simulink model "MOSSE_HDL_HIL_final"  (Simulink 8.1)
settings: Solver=FixedStepDiscrete  SolverMode=SingleTasking  StartTime=0.0  StopTime=20*30*640*360  RelTol=1e-3
InitFcn:
  | %% DSPBuilder Start
  | alt_dspbuilder_update_model(bdroot)
  | %% DSPBuilder End
  | K_shift = 4
  | 
  | ksize = 5
  | load('Gauss_coeff.mat')
  | tic
StopFcn:
  | % r = rcount.Data(:,:);
  | % w = wcount.Data(:,:);
  | % d = dout.Data(:,:);
  | % ir = read.Data(:,:);
  | % iw = write.Data(:,:);
  | % z = double([ir iw d r w]');
  | %logic_analyzer
  | toc
undefined symbols (not defined in the file or in its folder): gray, psr, source_1, source_2, State_Machine, State_Transition_Table1
libraries: allblocks_alteradspbuilder2 x75, hdldemolib x2, dspsigattribs x2, dspmtrx3 x2, visionsinks x1, visiontextngfix x1, dspvision x1
(part 1 of 2)
settings Model: FPTRunName=FPA_Reference  Creator=minimal  LastModifiedBy=minimal
settings DataIOCC: SignalLoggingSaveFormat=Dataset
settings OptimizationCC: ExpressionDepthLimit=128
settings DebuggingCC: FcnCallInpInsideContextMsg=EnableAllAsError
settings HardwareCC: ProdHWDeviceType=ASIC/FPGA->ASIC/FPGA  TargetIntDivRoundTo=Zero  TargetEndianess=LittleEndian  TargetHWDeviceType=MATLAB Host  ProdEqTarget=off
settings GRTTargetCC: CombineOutputUpdateFcns=on  GRTInterface=off

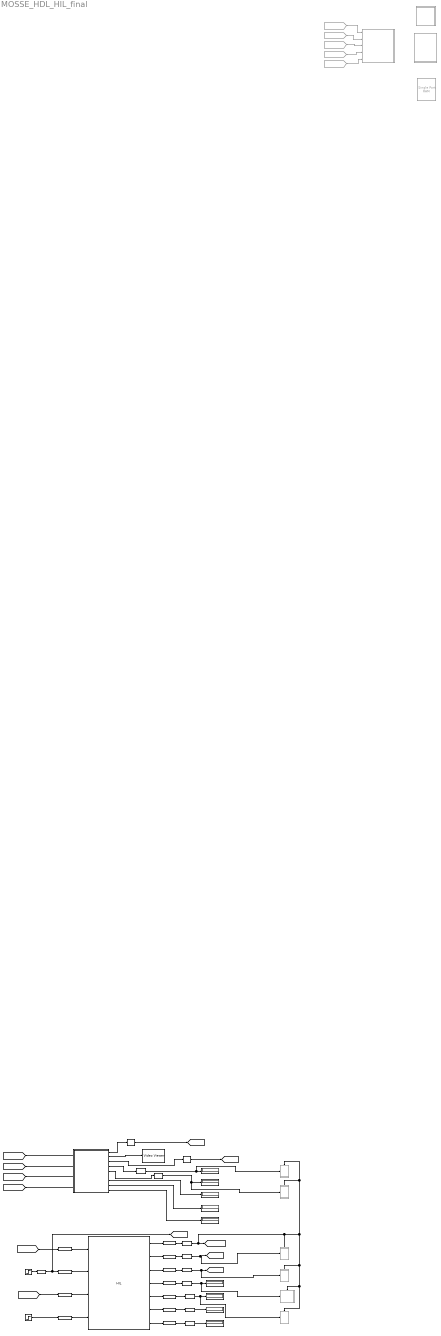
== system MOSSE_HDL_HIL_final ==
  Comp_Shift_Finish : allblocks_alteradspbuilder2/Output  iofile=d:\Project\AutoTracking\model\MOSSE_work\MOSSE_model\test\tb_MOSSE_HDL_HIL_final\MOSSE%5FHDL%5FHIL%5Ffinal_Comp%5FShift%5FFinish.capture  BusType=Single Bit  bwl=8  bwr=0  externalType=Simulink Fixed Point Type  PORTTYPE=Output  allowFloatingPointOverride=on  logOutputs=off
  DSP_Builder_Compute_PSR : Subsystem  Commented=on
  DSP_Builder_Compute_Shift : Subsystem  Commented=on
  Data Type Conversion{4,6..7,10} (4 alike) : DataTypeConversion  OutDataTypeStr=boolean
  Data Type Conversion11 : DataTypeConversion  OutDataTypeStr=int8
  Data Type Conversion12 : DataTypeConversion  OutDataTypeStr=int8
  Data Type Conversion13 : DataTypeConversion  OutDataTypeStr=uint16
  Data Type Conversion5 : DataTypeConversion  OutDataTypeStr=int16
  Data Type Conversion8 : DataTypeConversion  OutDataTypeStr=uint16
  Data Type Conversion9 : DataTypeConversion  OutDataTypeStr=uint16
  Delay2 : Delay  DelayLength=1  InitialCondition=0  SampleTime=1
  Delay3 : Delay  DelayLength=1  InitialCondition=0  SampleTime=1
  Display{,1..2,6} (4 alike) : Display
  Dx : allblocks_alteradspbuilder2/Output  iofile=d:\Project\AutoTracking\model\MOSSE_work\MOSSE_model\test\tb_MOSSE_HDL_HIL_final\MOSSE%5FHDL%5FHIL%5Ffinal_Dx.capture  BusType=Signed Integer  bwl=8  bwr=0  externalType=Simulink Fixed Point Type  PORTTYPE=Output  allowFloatingPointOverride=on  logOutputs=off
  Dy : allblocks_alteradspbuilder2/Output  iofile=d:\Project\AutoTracking\model\MOSSE_work\MOSSE_model\test\tb_MOSSE_HDL_HIL_final\MOSSE%5FHDL%5FHIL%5Ffinal_Dy.capture  BusType=Signed Integer  bwl=8  bwr=0  externalType=Simulink Fixed Point Type  PORTTYPE=Output  allowFloatingPointOverride=on  logOutputs=off
  Enable_Tracking : allblocks_alteradspbuilder2/Input  iofile=d:\Project\AutoTracking\model\MOSSE_work\MOSSE_model\test\tb_MOSSE_HDL_HIL_final\MOSSE%5FHDL%5FHIL%5Ffinal_Enable%5FTracking.salt  BusType=Single Bit  bwl=8  bwr=0  SpecifyClock=off  PORTTYPE=Input  externalType=Inferred  allowFloatingPointOverride=on  logOutputs=off
  Enable_Write : allblocks_alteradspbuilder2/Input  iofile=d:\Project\AutoTracking\model\MOSSE_work\MOSSE_model\test\tb_MOSSE_HDL_HIL_final\MOSSE%5FHDL%5FHIL%5Ffinal_Enable%5FWrite.salt  BusType=Single Bit  bwl=8  bwr=0  SpecifyClock=off  PORTTYPE=Input  externalType=Inferred  allowFloatingPointOverride=on  logOutputs=off
  From38 : From  Commented=on  GotoTag=source_enb
  From39 : From  Commented=on  GotoTag=source1_enb
  From40 : From  Commented=on  GotoTag=source_control
  From41 : From  Commented=on  GotoTag=source_count_enb
  From42 : From  Commented=on  GotoTag=source_count_rst
  HIL : allblocks_alteradspbuilder2/HIL  entityName=MOSSE_HDL_code_gen_final  inNames=Input_image enable_tracking enable_write reset  inBwls="8  1  1  1  1  1"  inBwrs="0  0  0  0  0  0"  inTypes=u b b b  inDelayed="0  0  0  0"  outNames=comp_shift_finish dx dy max_index psr psr_check psr_finish  outBwls="1   8   8  13  16   1   1"  outBwrs="0  0  0  0  0  0  0"  outTypes=b s s u s b b  resetNames=aclr  InputCount=6  InputNames=Clock Input_image aclr enable_tracking enable_write reset  InputWidth="1  8  1  1  1  1"  InputRepresentation="0  0  0  0  0  0"  InputExport="2  0  3  0  0  0"  InputFPP="0  0  0  0  0  0"  OutputCount=7  OutputNames=comp_shift_finish dx dy max_index psr psr_check psr_finish  OutputWidth="1   8   8  13  16   1   1"  OutputRepresentation="0  1  1  0  1  0  0"  OutputExport="0  0  0  0  0  0  0"  OutputFPP="0  0  0  0  0  0  0"  JtagCable=1  JtagDevice=1  BurstMode=on  BurstLength=512  FrameMode=off  SOP=0  OutValid=0  QuartusProject=D:\Project\AutoTracking\model\MOSSE_work\MOSSE_model\test\MOSSE_HDL_code_gen_final_dspbuilder\MOSSE_HDL_code_gen_final.qpf  HilNewConfig=off  ClockPinLocation=K17  ClockPinSource=0  HilDeviceOnBoard=EP4CE115F29C7  DR_length=56  dspbuilder_reset=on  SLD_NODE_INFO=5167554  AssertSclrBeforeSimulation=1  SampleTime=0  dspb_ver=0  ResetLevel=0  JtagCableName=USB-Blaster [USB-0]  JtagDeviceName=@1: EP3C120/EP4CE115 (0x020F70DD)  ClockNames=Clock
  IFFT_res : hdldemolib/Single Port RAM  Commented=on  ram_size=12  dout_type=New data
  Input_image : allblocks_alteradspbuilder2/Input  iofile=d:\Project\AutoTracking\model\MOSSE_work\MOSSE_model\test\tb_MOSSE_HDL_HIL_final\MOSSE%5FHDL%5FHIL%5Ffinal_Input%5Fimage.salt  BusType=Unsigned Integer  bwl=8  bwr=0  SpecifyClock=off  PORTTYPE=Input  externalType=Inferred  allowFloatingPointOverride=on  logOutputs=off
  Reset : allblocks_alteradspbuilder2/Input  iofile=d:\Project\AutoTracking\model\MOSSE_work\MOSSE_model\test\tb_MOSSE_HDL_HIL_final\MOSSE%5FHDL%5FHIL%5Ffinal_Reset.salt  BusType=Single Bit  bwl=8  bwr=0  SpecifyClock=off  PORTTYPE=Input  externalType=Inferred  allowFloatingPointOverride=on  logOutputs=off
  Source : Subsystem  Commented=on
  Step : Step  Before=1  After=0  SampleTime=0
  Step1 : Step  SampleTime=0
  Subsystem : Subsystem  Commented=on
  Subsystem1 : Subsystem  Commented=on
  Subsystem2 : Subsystem  Commented=on
  Subsystem3 : Subsystem  Commented=on
  Subsystem4 : Subsystem  Commented=on
  Subsystem5 : Subsystem  Commented=on
  Video Viewer2 : visionsinks/Video Viewer  inputType=Obsolete7b  imagePorts=One multidimensional signal  useColorMap=off  colormapValue=gray(256)  specRange=off  minInputVal=0  maxInputVal=255  FigPos=[321 948 1218 708]  AxisZoom=on  trueSizedOnce=off  OpenAtMdlStart=on  DefaultConfigurationName=vipscopes.VideoViewerScopeCfg
  Video_TestBench1 : Subsystem
  addr_x : Display
  addr_y : Display
  frame_num : Display
  max_index : allblocks_alteradspbuilder2/Output  iofile=d:\Project\AutoTracking\model\MOSSE_work\MOSSE_model\test\tb_MOSSE_HDL_HIL_final\MOSSE%5FHDL%5FHIL%5Ffinal_max%5Findex.capture  BusType=Unsigned Integer  bwl=13  bwr=0  externalType=Simulink Fixed Point Type  PORTTYPE=Output  allowFloatingPointOverride=on  logOutputs=off
  "psr " : allblocks_alteradspbuilder2/Output  iofile=d:\Project\AutoTracking\model\MOSSE_work\MOSSE_model\test\tb_MOSSE_HDL_HIL_final\MOSSE%5FHDL%5FHIL%5Ffinal_psr%0A.capture  BusType=Signed Integer  bwl=16  bwr=0  externalType=Simulink Fixed Point Type  PORTTYPE=Output  allowFloatingPointOverride=on  logOutputs=off
  psr_check : allblocks_alteradspbuilder2/Output  iofile=d:\Project\AutoTracking\model\MOSSE_work\MOSSE_model\test\tb_MOSSE_HDL_HIL_final\MOSSE%5FHDL%5FHIL%5Ffinal_psr%5Fcheck.capture  BusType=Single Bit  bwl=8  bwr=0  externalType=Simulink Fixed Point Type  PORTTYPE=Output  allowFloatingPointOverride=on  logOutputs=off
  psr_finish : allblocks_alteradspbuilder2/Output  iofile=d:\Project\AutoTracking\model\MOSSE_work\MOSSE_model\test\tb_MOSSE_HDL_HIL_final\MOSSE%5FHDL%5FHIL%5Ffinal_psr%5Ffinish.capture  BusType=Single Bit  bwl=8  bwr=0  externalType=Simulink Fixed Point Type  PORTTYPE=Output  allowFloatingPointOverride=on  logOutputs=off
  x : Display
  y : Display
  wires:
  From40/1 -> Source/1(source_control)
  From38/1 -> Source/2(source_enb)
  From42/1 -> Source/3(source_count_rst)
  From41/1 -> Source/4(source_count_enb)
  From39/1 -> Source/5(source1_enb)
  Data Type Conversion10/1 -> Subsystem/Enable, Subsystem2/Enable, Subsystem3/Enable, Subsystem1/Enable, Subsystem5/Enable, Subsystem4/Enable, [comp_shift_finish]
  Step/1 -> Reset/1
  Input_image/1 -> HIL/1
  Reset/1 -> HIL/4
  HIL/1 -> Comp_Shift_Finish/1
  HIL/2 -> Dx/1
  HIL/3 -> Dy/1
  [input_image] -> Input_image/1
  HIL/4 -> max_index/1
  HIL/6 -> psr_check/1
  Video_TestBench1/2(video_viewer) -> Video Viewer2/1
  Video_TestBench1/1(enable_write) -> Delay2/1
  Video_TestBench1/3(serialized_data) -> Delay3/1
  Delay3/1 -> [input_image]
  Delay2/1 -> [enable_write]
  [enable_tracking] -> Video_TestBench1/1(en)
  [comp_shift_finish] -> Video_TestBench1/4(comp_shift_finish)
  [dx] -> Video_TestBench1/2(dx)
  [dy] -> Video_TestBench1/3(dy)
  "psr "/1 -> Data Type Conversion5/1
  Data Type Conversion5/1 -> Subsystem2/1(psr), Display1/1
  psr_check/1 -> Data Type Conversion4/1
  Data Type Conversion4/1 -> Display/1
  psr_finish/1 -> Data Type Conversion6/1
  Data Type Conversion6/1 -> Display2/1
  HIL/7 -> psr_finish/1
  HIL/5 -> "psr "/1
  Video_TestBench1/7(frame_num) -> frame_num/1
  Data Type Conversion8/1 -> Subsystem4/1(addr_x), x/1
  Data Type Conversion9/1 -> Subsystem5/1(addr_y), y/1
  Video_TestBench1/8(addr_x) -> addr_x/1
  Video_TestBench1/9(addr_y) -> addr_y/1
  Enable_Tracking/1 -> HIL/2
  Data Type Conversion7/1 -> [enable_tracking], Enable_Tracking/1
  Step1/1 -> Data Type Conversion7/1
  [enable_write] -> Enable_Write/1
  Enable_Write/1 -> HIL/3
  Video_TestBench1/4(x) -> Data Type Conversion8/1
  Video_TestBench1/5(y) -> Data Type Conversion9/1
  Comp_Shift_Finish/1 -> Data Type Conversion10/1
  Data Type Conversion11/1 -> [dx], Subsystem/1(dx)
  Dx/1 -> Data Type Conversion11/1
  Dy/1 -> Data Type Conversion12/1
  Data Type Conversion12/1 -> [dy], Subsystem1/1(dy)
  max_index/1 -> Data Type Conversion13/1
  Data Type Conversion13/1 -> Display6/1, Subsystem3/1(max_index)

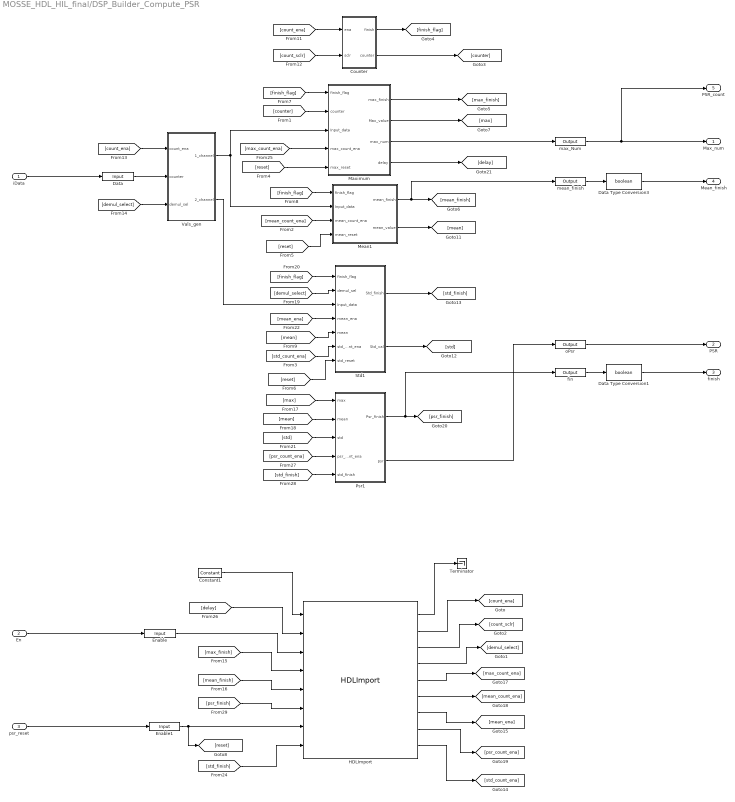
== system MOSSE_HDL_HIL_final/DSP_Builder_Compute_PSR ==
  iData : Inport
  En : Inport  Port=2
  psr_reset : Inport  Port=3
  Constant1 : allblocks_alteradspbuilder2/Constant  mask_cst=1  BusType=Single Bit  bwl=8  bwr=0  roundMode=Truncate  satMode=Wrap  SpecifyClock=off  allowFloatingPointOverride=on  logOutputs=off  logFile=d:\Project\AutoTracking\model\MOSSE_work\MOSSE_model\MOSSE_Final_models\tb_MOSSE_HDL_final\MOSSE%5FHDL%5Ffinal_DSP%5FBuilder%5FCompute%5FPSR_Constant1.fixedpointlog
  Counter : Subsystem
  Data : allblocks_alteradspbuilder2/Input  iofile=d:\Project\AutoTracking\model\MOSSE_work\MOSSE_model\MOSSE_Final_models\tb_MOSSE_HDL_final\MOSSE%5FHDL%5Ffinal_DSP%5FBuilder%5FCompute%5FPSR_Data.salt  BusType=Signed Integer  bwl=16  bwr=0  SpecifyClock=off  PORTTYPE=Input  externalType=Inferred  allowFloatingPointOverride=on  logOutputs=off
  Data Type Conversion1 : DataTypeConversion  OutDataTypeStr=boolean
  Data Type Conversion3 : DataTypeConversion  OutDataTypeStr=boolean
  Enable : allblocks_alteradspbuilder2/Input  iofile=d:\Project\AutoTracking\model\MOSSE_work\MOSSE_model\MOSSE_Final_models\tb_MOSSE_HDL_final\MOSSE%5FHDL%5Ffinal_DSP%5FBuilder%5FCompute%5FPSR_Enable.salt  BusType=Single Bit  bwl=16  bwr=0  SpecifyClock=off  PORTTYPE=Input  externalType=Inferred  allowFloatingPointOverride=on  logOutputs=off
  Enable1 : allblocks_alteradspbuilder2/Input  iofile=d:\Project\AutoTracking\model\MOSSE_work\MOSSE_model\MOSSE_Final_models\tb_MOSSE_HDL_final\MOSSE%5FHDL%5Ffinal_DSP%5FBuilder%5FCompute%5FPSR_Enable1.salt  BusType=Single Bit  bwl=16  bwr=0  SpecifyClock=off  PORTTYPE=Input  externalType=Inferred  allowFloatingPointOverride=on  logOutputs=off
  HDLImport : allblocks_alteradspbuilder2/HDLImport  entityName=State_Machine_import  inNames=clk_enable delay enable_in max_finish mean_finish psr_finish reset std_finish  inBwls=1 1 1 1 1 1 1 1  inBwrs="0  0  0  0  0  0  0  0"  inTypes=b b b b b b b b  inDelayed="0  0  0  0  0  0  0  0"  outNames=ce_out count_ena count_sclr demul_select max_count_ena mean_count_ena mean_ena psr_count_ena std_count_ena  outBwls=1 1 1 1 1 1 1 1 1  outBwrs="0  0  0  0  0  0  0  0  0"  outTypes=b b b b b b b b b  xmlmapfile=C:\altera\13.0\quartus\dsp_builder\lib\SimgenCMap.xml  vofile=DSPBuilder_MOSSE_HDL_final_import\State_Machine.vo  src_file=psr\State_Machine.v;psr\State_Transition_Table1.v;  TopLevelName=State_Machine  UseQPF=0  n_input_port=8  n_output_port=9  array_clocks=clk  use_systemC_model=off  is_megacore=off  use_dynamic_feedthrough_data=off  use_alphabetical_port_ordering=on  allowFloatingPointOverride=off
  Maximum : Subsystem
  Mean1 : Subsystem
  Psr1 : Subsystem
  Std1 : Subsystem
  Terminator : Terminator
  Vals_gen : Subsystem
  fin : allblocks_alteradspbuilder2/Output  iofile=d:\Project\AutoTracking\model\MOSSE_work\MOSSE_model\MOSSE_Final_models\tb_MOSSE_HDL_final\MOSSE%5FHDL%5Ffinal_DSP%5FBuilder%5FCompute%5FPSR_fin.capture  BusType=Single Bit  bwl=32  bwr=0  externalType=Simulink Fixed Point Type  PORTTYPE=Output  allowFloatingPointOverride=on  logOutputs=off
  max_Num : allblocks_alteradspbuilder2/Output  iofile=d:\Project\AutoTracking\model\MOSSE_work\MOSSE_model\MOSSE_Final_models\tb_MOSSE_HDL_final\MOSSE%5FHDL%5Ffinal_DSP%5FBuilder%5FCompute%5FPSR_max%5FNum.capture  BusType=Signed Integer  bwl=16  bwr=0  externalType=Simulink Fixed Point Type  PORTTYPE=Output  allowFloatingPointOverride=on  logOutputs=off
  mean_finish : allblocks_alteradspbuilder2/Output  iofile=d:\Project\AutoTracking\model\MOSSE_work\MOSSE_model\MOSSE_Final_models\tb_MOSSE_HDL_final\MOSSE%5FHDL%5Ffinal_DSP%5FBuilder%5FCompute%5FPSR_mean%5Ffinish.capture  BusType=Single Bit  bwl=16  bwr=0  externalType=Simulink Fixed Point Type  PORTTYPE=Output  allowFloatingPointOverride=on  logOutputs=off
  oPsr : allblocks_alteradspbuilder2/Output  iofile=d:\Project\AutoTracking\model\MOSSE_work\MOSSE_model\MOSSE_Final_models\tb_MOSSE_HDL_final\MOSSE%5FHDL%5Ffinal_DSP%5FBuilder%5FCompute%5FPSR_oPsr.capture  BusType=Signed Integer  bwl=32  bwr=0  externalType=Simulink Fixed Point Type  PORTTYPE=Output  allowFloatingPointOverride=on  logOutputs=off
  Max_num : Outport
  PSR : Outport  Port=2
  finish : Outport  Port=3
  Mean_finish : Outport  Port=4
  PSR_count : Outport  Port=5
  wires:
  [demul_select] -> Std1/2(demul_sel)
  Data/1 -> Vals_gen/2(counter)
  [demul_select] -> Vals_gen/3(demul_sel)
  Vals_gen/2(2_channel) -> Std1/3(Input_data)
  [finish_flag] -> Std1/1(finish_flag)
  Std1/1(Std_finish) -> [std_finish]
  Mean1/2(mean_value) -> [mean]
  max_Num/1 -> PSR_count/1, Max_num/1
  Maximum/2(Max_value) -> [max]
  [mean] -> Std1/5(mean)
  [mean_ena] -> Std1/4(mean_ena)
  [max] -> Psr1/1(max)
  Maximum/4(delay) -> [delay]
  HDLImport/1 -> Terminator/1
  Constant1/1 -> HDLImport/1
  [psr_finish] -> HDLImport/6
  [std_finish] -> HDLImport/8
  [mean_finish] -> HDLImport/5
  [max_finish] -> HDLImport/4
  [delay] -> HDLImport/2
  Mean1/1(mean_finish) -> mean_finish/1, [mean_finish]
  oPsr/1 -> PSR/1
  [count_ena] -> Vals_gen/1(count_ena)
  Psr1/1(Psr_finish) -> fin/1, [psr_finish]
  Vals_gen/1(1_channel) -> Maximum/3(Input_data), Mean1/2(Input_data)
  [mean_count_ena] -> Mean1/3(mean_count_ena)
  Counter/1(finish) -> [finish_flag]
  Maximum/1(max_finish) -> [max_finish]
  [counter] -> Maximum/2(counter)
  [finish_flag] -> Maximum/1(finish_flag)
  [finish_flag] -> Mean1/1(finish_flag)
  [count_ena] -> Counter/1(ena)
  [count_sclr] -> Counter/2(sclr)
  [std_finish] -> Psr1/5(std_finish)
  Psr1/2(psr) -> oPsr/1
  [mean] -> Psr1/2(mean)
  [std] -> Psr1/3(std)
  Std1/2(Std_val) -> [std]
  [std_count_ena] -> Std1/6(std_count_ena)
  [psr_count_ena] -> Psr1/4(psr_count_ena)
  [max_count_ena] -> Maximum/4(max_count_ena)
  HDLImport/3 -> [count_sclr]
  HDLImport/2 -> [count_ena]
  HDLImport/6 -> [mean_count_ena]
  Enable/1 -> HDLImport/3
  HDLImport/4 -> [demul_select]
  HDLImport/5 -> [max_count_ena]
  HDLImport/7 -> [mean_ena]
  HDLImport/8 -> [psr_count_ena]
  HDLImport/9 -> [std_count_ena]
  Counter/2(counter) -> [counter]
  En/1 -> Enable/1
  iData/1 -> Data/1
  psr_reset/1 -> Enable1/1
  Enable1/1 -> [reset], HDLImport/7
  mean_finish/1 -> Data Type Conversion3/1
  fin/1 -> Data Type Conversion1/1
  Data Type Conversion1/1 -> finish/1
  Data Type Conversion3/1 -> Mean_finish/1
  [reset] -> Maximum/5(max_reset)
  [reset] -> Mean1/4(mean_reset)
  [reset] -> Std1/7(std_reset)
  Maximum/3(max_num) -> max_Num/1

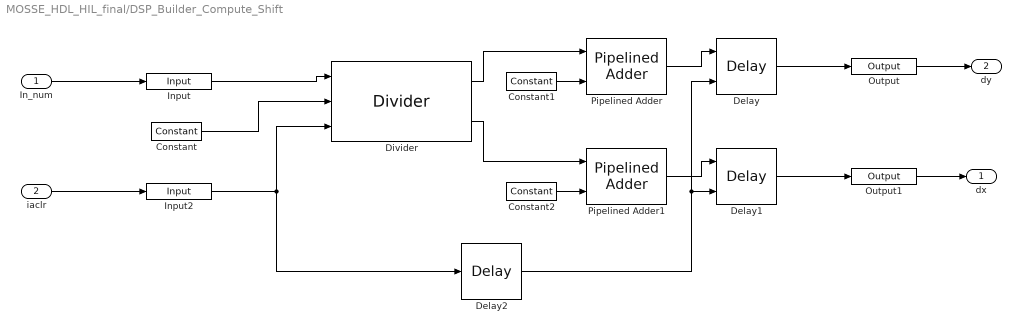
== system MOSSE_HDL_HIL_final/DSP_Builder_Compute_Shift ==
  In_num : Inport
  iaclr : Inport  Port=2
  Constant : allblocks_alteradspbuilder2/Constant  mask_cst=64  BusType=Unsigned Integer  bwl=8  bwr=0  roundMode=Truncate  satMode=Wrap  SpecifyClock=off  allowFloatingPointOverride=on  logOutputs=off  logFile=C:\Workspace\Autotracking\MOSSE_model\tb_MOSSE_HDL_final\MOSSE%5FHDL%5Ffinal_DSP%5FBuilder%5FCompute%5FShift_Constant.fixedpointlog
  Constant1 : allblocks_alteradspbuilder2/Constant  mask_cst=31  BusType=Signed Integer  bwl=8  bwr=0  roundMode=Truncate  satMode=Wrap  SpecifyClock=off  allowFloatingPointOverride=on  logOutputs=off  logFile=C:\Workspace\Autotracking\MOSSE_model\tb_MOSSE_HDL_final\MOSSE%5FHDL%5Ffinal_DSP%5FBuilder%5FCompute%5FShift_Constant1.fixedpointlog
  Constant2 : allblocks_alteradspbuilder2/Constant  mask_cst=32  BusType=Signed Integer  bwl=8  bwr=0  roundMode=Truncate  satMode=Wrap  SpecifyClock=off  allowFloatingPointOverride=on  logOutputs=off  logFile=C:\Workspace\Autotracking\MOSSE_model\tb_MOSSE_HDL_final\MOSSE%5FHDL%5Ffinal_DSP%5FBuilder%5FCompute%5FShift_Constant2.fixedpointlog
  Delay : allblocks_alteradspbuilder2/Delay  pipeline=1  pipeline_display=1  ClockPhase=1  use_ena=off  use_sclr=on  allowFloatingPointOverride=on  logOutputs=off  logFile=C:\Workspace\Autotracking\MOSSE_model\tb_MOSSE_HDL_final\MOSSE%5FHDL%5Ffinal_DSP%5FBuilder%5FCompute%5FShift_Delay.fixedpointlog  use_init=off  reset_value=1
  Delay1 : allblocks_alteradspbuilder2/Delay  pipeline=1  pipeline_display=1  ClockPhase=1  use_ena=off  use_sclr=on  allowFloatingPointOverride=on  logOutputs=off  logFile=C:\Workspace\Autotracking\MOSSE_model\tb_MOSSE_HDL_final\MOSSE%5FHDL%5Ffinal_DSP%5FBuilder%5FCompute%5FShift_Delay1.fixedpointlog  use_init=off  reset_value=1
  Delay2 : allblocks_alteradspbuilder2/Delay  pipeline=1  pipeline_display=1  ClockPhase=1  use_ena=off  use_sclr=off  allowFloatingPointOverride=on  logOutputs=off  logFile=C:\Workspace\Autotracking\MOSSE_model\tb_MOSSE_HDL_final\MOSSE%5FHDL%5Ffinal_DSP%5FBuilder%5FCompute%5FShift_Delay2.fixedpointlog  use_init=off  reset_value=1
  Divider : allblocks_alteradspbuilder2/Divider  BusType=Unsigned Integer  bwl=12  bwr=0  pipeline=1  pipeline_display=1  use_ena=off  use_aclr=on
  Input : allblocks_alteradspbuilder2/Input  iofile=C:\Workspace\Autotracking\MOSSE_model\tb_MOSSE_HDL_final\MOSSE%5FHDL%5Ffinal_DSP%5FBuilder%5FCompute%5FShift_Input.salt  BusType=Unsigned Integer  bwl=12  bwr=0  SpecifyClock=off  PORTTYPE=Input  externalType=Inferred  allowFloatingPointOverride=on  logOutputs=off
  Input2 : allblocks_alteradspbuilder2/Input  iofile=C:\Workspace\Autotracking\MOSSE_model\tb_MOSSE_HDL_final\MOSSE%5FHDL%5Ffinal_DSP%5FBuilder%5FCompute%5FShift_Input2.salt  BusType=Single Bit  bwl=12  bwr=0  SpecifyClock=off  PORTTYPE=Input  externalType=Inferred  allowFloatingPointOverride=on  logOutputs=off
  Output : allblocks_alteradspbuilder2/Output  iofile=C:\Workspace\Autotracking\MOSSE_model\tb_MOSSE_HDL_final\MOSSE%5FHDL%5Ffinal_DSP%5FBuilder%5FCompute%5FShift_Output.capture  BusType=Signed Integer  bwl=8  bwr=0  externalType=Simulink Fixed Point Type  PORTTYPE=Output  allowFloatingPointOverride=on  logOutputs=off
  Output1 : allblocks_alteradspbuilder2/Output  iofile=C:\Workspace\Autotracking\MOSSE_model\tb_MOSSE_HDL_final\MOSSE%5FHDL%5Ffinal_DSP%5FBuilder%5FCompute%5FShift_Output1.capture  BusType=Signed Integer  bwl=8  bwr=0  externalType=Simulink Fixed Point Type  PORTTYPE=Output  allowFloatingPointOverride=on  logOutputs=off
  Pipelined Adder : allblocks_alteradspbuilder2/Pipelined Adder  BusType=Signed Integer  bwl=12  bwr=0  pipeline=0  pipeline_display=0  AddSubDirection=SUB  use_cin=off  use_ovl=off  use_addsub=off  use_ena=off  use_aclr=off  or_aclr_inputs=on
  Pipelined Adder1 : allblocks_alteradspbuilder2/Pipelined Adder  BusType=Signed Integer  bwl=12  bwr=0  pipeline=0  pipeline_display=0  AddSubDirection=SUB  use_cin=off  use_ovl=off  use_addsub=off  use_ena=off  use_aclr=off  or_aclr_inputs=on
  dx : Outport
  dy : Outport  Port=2
  wires:
  Input/1 -> Divider/1
  Constant/1 -> Divider/2
  In_num/1 -> Input/1
  Output1/1 -> dx/1
  Output/1 -> dy/1
  Divider/1 -> Pipelined Adder/1
  Constant2/1 -> Pipelined Adder1/2
  Pipelined Adder/1 -> Delay/1
  Delay/1 -> Output/1
  Pipelined Adder1/1 -> Delay1/1
  Delay1/1 -> Output1/1
  Divider/2 -> Pipelined Adder1/1
  iaclr/1 -> Input2/1
  Input2/1 -> Delay2/1, Divider/3
  Constant1/1 -> Pipelined Adder/2
  Delay2/1 -> Delay/2, Delay1/2

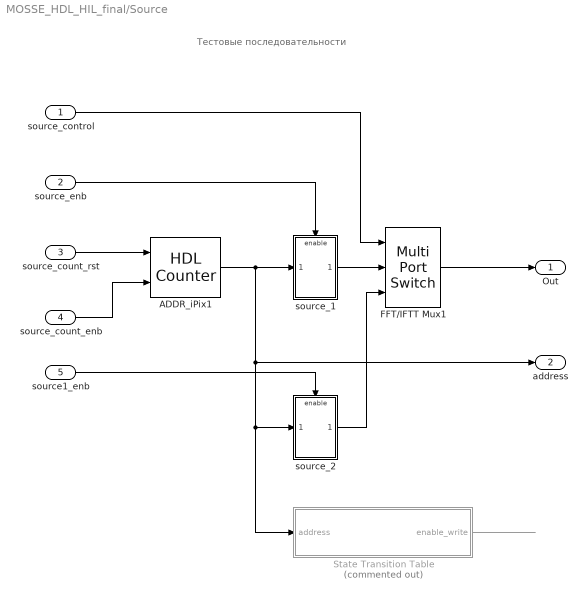
== system MOSSE_HDL_HIL_final/Source ==
  note: Тестовые последовательности
  source_control : Inport
  source_enb : Inport  Port=2
  source_count_rst : Inport  Port=3
  source_count_enb : Inport  Port=4
  source1_enb : Inport  Port=5
  ADDR_iPix1 : hdldemolib/HDL Counter  CountType=Free running  CountInit=0  CountStep=1  CountMax=100  CountFromType=Initial value  CountFrom=0  CountResetPort=on  CountLoadPort=off  CountEnbPort=on  CountDirPort=off  CountDataType=Unsigned  CountWordLen=32  CountFracLen=0  CountSampTime=1
  FFT/IFTT Mux1 : MultiPortSwitch  DataPortOrder=Zero-based contiguous  Inputs=2  zeroidx=on  OutDataTypeStr=fixdt(1,24,0)  SampleTime=1
  State Transition Table : State Transition Table  Commented=on  TreatAsAtomicUnit=on
  source_1 : Subsystem
  source_2 : Subsystem
  Out : Outport
  address : Outport  Port=2
  wires:
  ADDR_iPix1/1 -> address/1, State Transition Table/1(address), source_2/1(In1), source_1/1(In1)
  source_enb/1 -> source_1/Enable
  source1_enb/1 -> source_2/Enable
  source_count_enb/1 -> ADDR_iPix1/2
  FFT/IFTT Mux1/1 -> Out/1
  source_count_rst/1 -> ADDR_iPix1/1
  source_1/1(Out1) -> FFT/IFTT Mux1/2
  source_control/1 -> FFT/IFTT Mux1/1
  source_2/1(Out1) -> FFT/IFTT Mux1/3
  State Transition Table/1(enable_write) -> ?

== system MOSSE_HDL_HIL_final/Subsystem ==
  dx : Inport
  Enable : EnablePort
  To Workspace : ToWorkspace  VariableName=dx  SampleTime=-1
  wires:
  dx/1 -> To Workspace/1

== system MOSSE_HDL_HIL_final/Subsystem1 ==
  dy : Inport
  Enable : EnablePort
  To Workspace : ToWorkspace  VariableName=dy  SampleTime=-1
  wires:
  dy/1 -> To Workspace/1

== system MOSSE_HDL_HIL_final/Subsystem2 ==
  psr : Inport
  Enable : EnablePort
  To Workspace : ToWorkspace  VariableName=psr  SampleTime=-1
  wires:
  psr/1 -> To Workspace/1

== system MOSSE_HDL_HIL_final/Subsystem3 ==
  max_index : Inport
  Enable : EnablePort
  To Workspace : ToWorkspace  VariableName=max_index  SampleTime=-1
  wires:
  max_index/1 -> To Workspace/1

== system MOSSE_HDL_HIL_final/Subsystem4 ==
  addr_x : Inport
  Enable : EnablePort
  To Workspace : ToWorkspace  VariableName=addr_x  SampleTime=-1
  wires:
  addr_x/1 -> To Workspace/1

== system MOSSE_HDL_HIL_final/Subsystem5 ==
  addr_y : Inport
  Enable : EnablePort
  To Workspace : ToWorkspace  VariableName=addr_y  SampleTime=-1
  wires:
  addr_y/1 -> To Workspace/1

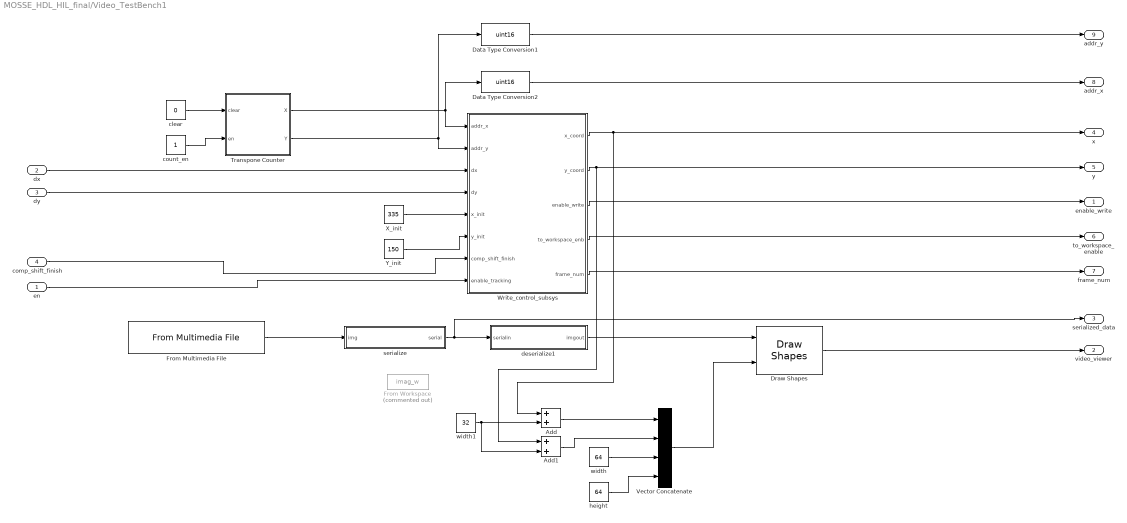
== system MOSSE_HDL_HIL_final/Video_TestBench1 ==
  en : Inport
  dx : Inport  Port=2
  dy : Inport  Port=3
  comp_shift_finish : Inport  Port=4
  Add : Sum  AccumDataTypeStr=uint16
  Add1 : Sum  AccumDataTypeStr=uint16
  Data Type Conversion1 : DataTypeConversion  OutDataTypeStr=uint16
  Data Type Conversion2 : DataTypeConversion  OutDataTypeStr=uint16
  Draw Shapes : visiontextngfix/Draw Shapes  shape=Rectangles  fill=off  fillClrSource=Specify via dialog  display=User-specified value  intensity=200  color=[255]  opacity=0.6  viewport=Entire image  antialiasing=off  inType=Obsolete  imagePorts=One multidimensional signal  prodOutputMode=Binary point scaling  prodOutputWordLength=32  prodOutputFracLength=14  memoryMode=Specify word length  memoryWordLength=16  memoryFracLength=15  roundingMode=Floor  overflowMode=off
  From Workspace : FromWorkspace  Commented=on  VariableName=imag_w  SampleTime=1
  From Multimedia File : dspvision/From Multimedia File  inputFilename=D:\Project\AutoTracking\model\MOSSE_work\MOSSE_model\test\test_video_2.avi  loop=on  numPlays=inf  outputStreams=Video only  videoDataType=uint8  audioDataType=int16  inheritSampleTime=off  userDefinedSampleTime=640*360  noAudioOutput=off  isIntensityVideo=off  fourcc=Intensity  colorVideoFormat=One multidimensional signal  outputEOF=off  dataOrg=Column-major  audioFrameSize=1024  computeAudioFrameSize=off  outSamplingMode=Sample based
  Transpone Counter : MATLAB Function
  Vector Concatenate : Concatenate  NumInputs=4
  Write_control_subsys : Subsystem
  X_init : Constant  Value=335  OutDataTypeStr=uint16
  Y_init : Constant  Value=150  OutDataTypeStr=uint16
  clear : Constant  Value=0  OutDataTypeStr=boolean
  count_en : Constant  OutDataTypeStr=boolean
  deserialize1 : Subsystem
  height : Constant  Value=64  OutDataTypeStr=uint16
  serialize : Subsystem
  width : Constant  Value=64  OutDataTypeStr=uint16
  width1 : Constant  Value=32  OutDataTypeStr=uint16
  enable_write : Outport
  video_viewer : Outport  Port=2
  serialized_data : Outport  Port=3
  x : Outport  Port=4
  y : Outport  Port=5
  to_workspace_enable : Outport  Port=6
  frame_num : Outport  Port=7
  addr_x : Outport  Port=8
  addr_y : Outport  Port=9
  wires:
  From Multimedia File/1 -> serialize/1(img)
  deserialize1/1(imgout) -> Draw Shapes/1
  serialize/1(serial) -> deserialize1/1(serialin), serialized_data/1
  Transpone Counter/2(Y) -> Write_control_subsys/2(addr_y), Data Type Conversion1/1
  Transpone Counter/1(X) -> Write_control_subsys/1(addr_x), Data Type Conversion2/1
  count_en/1 -> Transpone Counter/2(en)
  clear/1 -> Transpone Counter/1(clear)
  en/1 -> Write_control_subsys/8(enable_tracking)
  Draw Shapes/1 -> video_viewer/1
  width/1 -> Vector Concatenate/3
  height/1 -> Vector Concatenate/4
  Vector Concatenate/1 -> Draw Shapes/2
  Add1/1 -> Vector Concatenate/2
  Add/1 -> Vector Concatenate/1
  Data Type Conversion1/1 -> addr_y/1
  Data Type Conversion2/1 -> addr_x/1
  width1/1 -> Add/2, Add1/2
  Write_control_subsys/1(x_coord) -> x/1, Add/1
  Write_control_subsys/2(y_coord) -> y/1, Add1/1
  dx/1 -> Write_control_subsys/3(dx)
  X_init/1 -> Write_control_subsys/5(x_init)
  dy/1 -> Write_control_subsys/4(dy)
  comp_shift_finish/1 -> Write_control_subsys/7(comp_shift_finish)
  Write_control_subsys/3(enable_write) -> enable_write/1
  Write_control_subsys/4(to_workspace_enb) -> to_workspace_enable/1
  Write_control_subsys/5(frame_num) -> frame_num/1
  Y_init/1 -> Write_control_subsys/6(y_init)

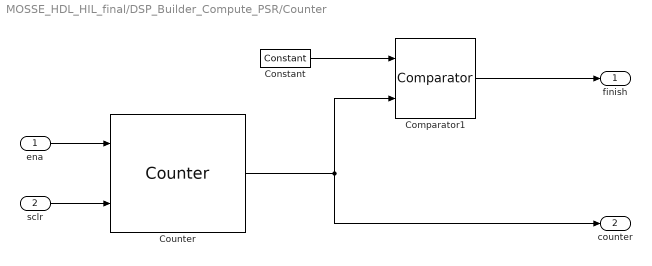
== system MOSSE_HDL_HIL_final/DSP_Builder_Compute_PSR/Counter ==
  ena : Inport
  sclr : Inport  Port=2
  Comparator1 : allblocks_alteradspbuilder2/Comparator  direction=a == b  pipeline_display=0  allowFloatingPointOverride=on  logOutputs=off  logFile=d:\Project\AutoTracking\model\MOSSE_work\MOSSE_model\MOSSE_Final_models\tb_MOSSE_HDL_final\MOSSE%5FHDL%5Ffinal_DSP%5FBuilder%5FCompute%5FPSR_Counter_Comparator1.fixedpointlog
  Constant : allblocks_alteradspbuilder2/Constant  mask_cst=4095  BusType=Unsigned Integer  bwl=16  bwr=0  roundMode=Truncate  satMode=Wrap  SpecifyClock=off  allowFloatingPointOverride=on  logOutputs=off  logFile=d:\Project\AutoTracking\model\MOSSE_work\MOSSE_model\MOSSE_Final_models\tb_MOSSE_HDL_final\MOSSE%5FHDL%5Ffinal_DSP%5FBuilder%5FCompute%5FPSR_Counter_Constant.fixedpointlog
  Counter : allblocks_alteradspbuilder2/Counter  BusType=Unsigned Integer  bwl=16  bwr=0  use_modulo=on  modulo=4100  SpecifyClock=off  direction=Increment  use_sload=off  use_sset=off  svalue=1  use_clk_ena=off  use_ena=on  use_sclr=on  pipeline_display=1
  finish : Outport
  counter : Outport  Port=2
  wires:
  Constant/1 -> Comparator1/1
  Counter/1 -> counter/1, Comparator1/2
  Comparator1/1 -> finish/1
  sclr/1 -> Counter/2
  ena/1 -> Counter/1

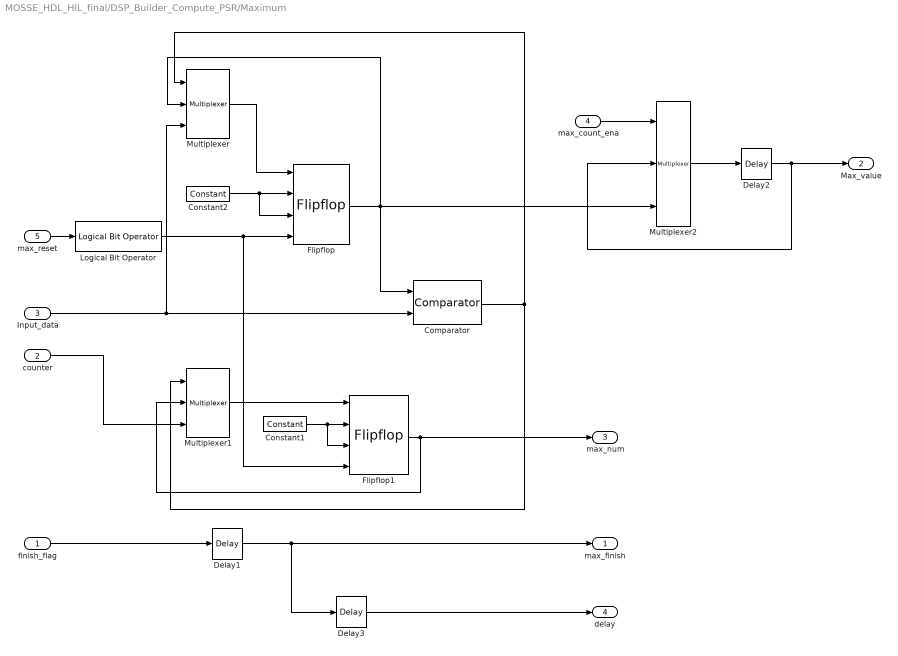
== system MOSSE_HDL_HIL_final/DSP_Builder_Compute_PSR/Maximum ==
  finish_flag : Inport
  counter : Inport  Port=2
  Input_data : Inport  Port=3
  max_count_ena : Inport  Port=4
  max_reset : Inport  Port=5
  Comparator : allblocks_alteradspbuilder2/Comparator  direction=a < b  pipeline_display=0  allowFloatingPointOverride=on  logOutputs=off  logFile=d:\Project\AutoTracking\model\MOSSE_work\MOSSE_model\MOSSE_Final_models\tb_MOSSE_HDL_final\MOSSE%5FHDL%5Ffinal_DSP%5FBuilder%5FCompute%5FPSR_Maximum_Comparator.fixedpointlog
  Constant1 : allblocks_alteradspbuilder2/Constant  mask_cst=1  BusType=Single Bit  bwl=24  bwr=0  roundMode=Truncate  satMode=Wrap  SpecifyClock=off  allowFloatingPointOverride=on  logOutputs=off  logFile=d:\Project\AutoTracking\model\MOSSE_work\MOSSE_model\MOSSE_Final_models\tb_MOSSE_HDL_final\MOSSE%5FHDL%5Ffinal_DSP%5FBuilder%5FCompute%5FPSR_Maximum_Constant1.fixedpointlog
  Constant2 : allblocks_alteradspbuilder2/Constant  mask_cst=1  BusType=Single Bit  bwl=24  bwr=0  roundMode=Truncate  satMode=Wrap  SpecifyClock=off  allowFloatingPointOverride=on  logOutputs=off  logFile=d:\Project\AutoTracking\model\MOSSE_work\MOSSE_model\MOSSE_Final_models\tb_MOSSE_HDL_final\MOSSE%5FHDL%5Ffinal_DSP%5FBuilder%5FCompute%5FPSR_Maximum_Constant2.fixedpointlog
  Delay1 : allblocks_alteradspbuilder2/Delay  pipeline=2  pipeline_display=2  ClockPhase=1  use_ena=off  use_sclr=off  allowFloatingPointOverride=on  logOutputs=off  logFile=d:\Project\AutoTracking\model\MOSSE_work\MOSSE_model\MOSSE_Final_models\tb_MOSSE_HDL_final\MOSSE%5FHDL%5Ffinal_DSP%5FBuilder%5FCompute%5FPSR_Maximum_Delay1.fixedpointlog  use_init=off  reset_value=1
  Delay2 : allblocks_alteradspbuilder2/Delay  pipeline=1  pipeline_display=1  ClockPhase=1  use_ena=off  use_sclr=off  allowFloatingPointOverride=on  logOutputs=off  logFile=d:\Project\AutoTracking\model\MOSSE_work\MOSSE_model\MOSSE_Final_models\tb_MOSSE_HDL_final\MOSSE%5FHDL%5Ffinal_DSP%5FBuilder%5FCompute%5FPSR_Maximum_Delay2.fixedpointlog  use_init=off  reset_value=1
  Delay3 : allblocks_alteradspbuilder2/Delay  pipeline=1  pipeline_display=1  ClockPhase=1  use_ena=off  use_sclr=off  allowFloatingPointOverride=on  logOutputs=off  logFile=d:\Project\AutoTracking\model\MOSSE_work\MOSSE_model\MOSSE_Final_models\tb_MOSSE_HDL_final\MOSSE%5FHDL%5Ffinal_DSP%5FBuilder%5FCompute%5FPSR_Maximum_Delay3.fixedpointlog  use_init=off  reset_value=1
  Flipflop : allblocks_alteradspbuilder2/Flipflop  mode=DFFE  BusType=Signed Integer  bwl=16  bwr=2  pipeline_display=1
  Flipflop1 : allblocks_alteradspbuilder2/Flipflop  mode=DFFE  BusType=Signed Integer  bwl=16  bwr=2  pipeline_display=1
  Logical Bit Operator : allblocks_alteradspbuilder2/Logical Bit Operator  LogicalOperator=NOT  user_inputs=2  pipeline_display=0
  Multiplexer : allblocks_alteradspbuilder2/Multiplexer  numInputs=2  pipeline=0  oneHot=off  pipeline_display=0  use_ena=off  use_aclr=off  allowFloatingPointOverride=on  logOutputs=off  logFile=d:\Project\AutoTracking\model\MOSSE_work\MOSSE_model\MOSSE_Final_models\tb_MOSSE_HDL_final\MOSSE%5FHDL%5Ffinal_DSP%5FBuilder%5FCompute%5FPSR_Maximum_Multiplexer.fixedpointlog
  Multiplexer1 : allblocks_alteradspbuilder2/Multiplexer  numInputs=2  pipeline=0  oneHot=off  pipeline_display=0  use_ena=off  use_aclr=off  allowFloatingPointOverride=on  logOutputs=off  logFile=d:\Project\AutoTracking\model\MOSSE_work\MOSSE_model\MOSSE_Final_models\tb_MOSSE_HDL_final\MOSSE%5FHDL%5Ffinal_DSP%5FBuilder%5FCompute%5FPSR_Maximum_Multiplexer1.fixedpointlog
  Multiplexer2 : allblocks_alteradspbuilder2/Multiplexer  numInputs=2  pipeline=0  oneHot=off  pipeline_display=0  use_ena=off  use_aclr=off  allowFloatingPointOverride=on  logOutputs=off  logFile=d:\Project\AutoTracking\model\MOSSE_work\MOSSE_model\MOSSE_Final_models\tb_MOSSE_HDL_final\MOSSE%5FHDL%5Ffinal_DSP%5FBuilder%5FCompute%5FPSR_Maximum_Multiplexer2.fixedpointlog
  max_finish : Outport
  Max_value : Outport  Port=2
  max_num : Outport  Port=3
  delay : Outport  Port=4
  wires:
  Comparator/1 -> Multiplexer/1, Multiplexer1/1
  Flipflop/1 -> Comparator/1, Multiplexer2/3, Multiplexer/2
  Multiplexer/1 -> Flipflop/1
  Constant2/1 -> Flipflop/3, Flipflop/2
  Input_data/1 -> Multiplexer/3, Comparator/2
  Flipflop1/1 -> max_num/1, Multiplexer1/2
  Multiplexer1/1 -> Flipflop1/1
  Constant1/1 -> Flipflop1/3, Flipflop1/2
  counter/1 -> Multiplexer1/3
  Delay1/1 -> max_finish/1, Delay3/1
  max_count_ena/1 -> Multiplexer2/1
  Multiplexer2/1 -> Delay2/1
  Delay2/1 -> Multiplexer2/2, Max_value/1
  Delay3/1 -> delay/1
  finish_flag/1 -> Delay1/1
  Logical Bit Operator/1 -> Flipflop1/4, Flipflop/4
  max_reset/1 -> Logical Bit Operator/1

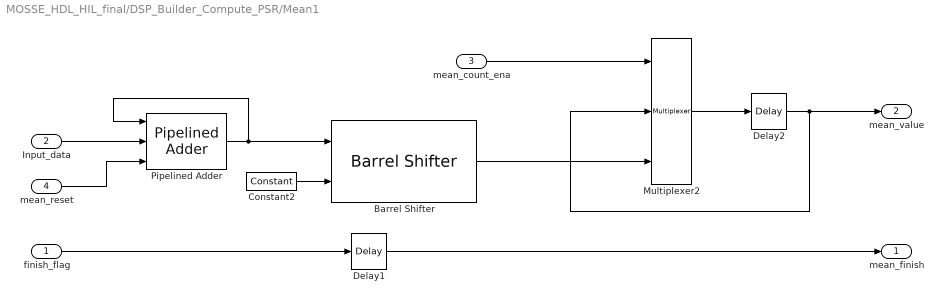
== system MOSSE_HDL_HIL_final/DSP_Builder_Compute_PSR/Mean1 ==
  finish_flag : Inport
  Input_data : Inport  Port=2
  mean_count_ena : Inport  Port=3
  mean_reset : Inport  Port=4
  Barrel Shifter : allblocks_alteradspbuilder2/Barrel Shifter  BusType=Signed Integer  bwl=32  bwr=8  pipeline=off  infer_distance=off  distance_length=4  ShiftDirection=Shift right  use_ena=off  use_aclr=off  UseDedicatedCircuitry=off  pipeline_display=0  allowFloatingPointOverride=on  logOutputs=off  logFile=d:\Project\AutoTracking\model\MOSSE_work\MOSSE_model\MOSSE_Final_models\tb_MOSSE_HDL_final\MOSSE%5FHDL%5Ffinal_DSP%5FBuilder%5FCompute%5FPSR_Mean1_Barrel+Shifter.fixedpointlog
  Constant2 : allblocks_alteradspbuilder2/Constant  mask_cst=12  BusType=Unsigned Integer  bwl=4  bwr=0  roundMode=Truncate  satMode=Wrap  SpecifyClock=off  allowFloatingPointOverride=on  logOutputs=off  logFile=d:\Project\AutoTracking\model\MOSSE_work\MOSSE_model\MOSSE_Final_models\tb_MOSSE_HDL_final\MOSSE%5FHDL%5Ffinal_DSP%5FBuilder%5FCompute%5FPSR_Mean1_Constant2.fixedpointlog
  Delay1 : allblocks_alteradspbuilder2/Delay  pipeline=1  pipeline_display=1  ClockPhase=1  use_ena=off  use_sclr=off  allowFloatingPointOverride=on  logOutputs=off  logFile=d:\Project\AutoTracking\model\MOSSE_work\MOSSE_model\MOSSE_Final_models\tb_MOSSE_HDL_final\MOSSE%5FHDL%5Ffinal_DSP%5FBuilder%5FCompute%5FPSR_Mean1_Delay1.fixedpointlog  use_init=off  reset_value=1
  Delay2 : allblocks_alteradspbuilder2/Delay  pipeline=1  pipeline_display=1  ClockPhase=1  use_ena=off  use_sclr=off  allowFloatingPointOverride=on  logOutputs=off  logFile=d:\Project\AutoTracking\model\MOSSE_work\MOSSE_model\MOSSE_Final_models\tb_MOSSE_HDL_final\MOSSE%5FHDL%5Ffinal_DSP%5FBuilder%5FCompute%5FPSR_Mean1_Delay2.fixedpointlog  use_init=off  reset_value=1
  Multiplexer2 : allblocks_alteradspbuilder2/Multiplexer  numInputs=2  pipeline=0  oneHot=off  pipeline_display=0  use_ena=off  use_aclr=off  allowFloatingPointOverride=on  logOutputs=off  logFile=d:\Project\AutoTracking\model\MOSSE_work\MOSSE_model\MOSSE_Final_models\tb_MOSSE_HDL_final\MOSSE%5FHDL%5Ffinal_DSP%5FBuilder%5FCompute%5FPSR_Mean1_Multiplexer2.fixedpointlog
  Pipelined Adder : allblocks_alteradspbuilder2/Pipelined Adder  BusType=Signed Integer  bwl=32  bwr=0  pipeline=1  pipeline_display=1  AddSubDirection=ADD  use_cin=off  use_ovl=off  use_addsub=off  use_ena=off  use_aclr=on  or_aclr_inputs=off
  mean_finish : Outport
  mean_value : Outport  Port=2
  wires:
  Constant2/1 -> Barrel Shifter/2
  Pipelined Adder/1 -> Pipelined Adder/1, Barrel Shifter/1
  Input_data/1 -> Pipelined Adder/2
  Barrel Shifter/1 -> Multiplexer2/3
  mean_count_ena/1 -> Multiplexer2/1
  Multiplexer2/1 -> Delay2/1
  Delay2/1 -> mean_value/1, Multiplexer2/2
  finish_flag/1 -> Delay1/1
  Delay1/1 -> mean_finish/1
  mean_reset/1 -> Pipelined Adder/3

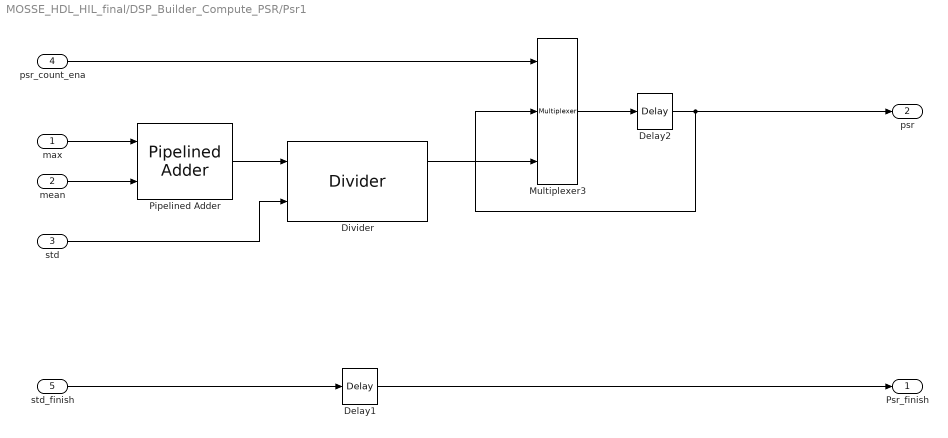
== system MOSSE_HDL_HIL_final/DSP_Builder_Compute_PSR/Psr1 ==
  max : Inport
  mean : Inport  Port=2
  std : Inport  Port=3
  psr_count_ena : Inport  Port=4
  std_finish : Inport  Port=5
  Delay1 : allblocks_alteradspbuilder2/Delay  pipeline=1  pipeline_display=1  ClockPhase=1  use_ena=off  use_sclr=off  allowFloatingPointOverride=on  logOutputs=off  logFile=d:\Project\AutoTracking\model\MOSSE_work\MOSSE_model\MOSSE_Final_models\tb_MOSSE_HDL_final\MOSSE%5FHDL%5Ffinal_DSP%5FBuilder%5FCompute%5FPSR_Psr1_Delay1.fixedpointlog  use_init=off  reset_value=1
  Delay2 : allblocks_alteradspbuilder2/Delay  pipeline=1  pipeline_display=1  ClockPhase=1  use_ena=off  use_sclr=off  allowFloatingPointOverride=on  logOutputs=off  logFile=d:\Project\AutoTracking\model\MOSSE_work\MOSSE_model\MOSSE_Final_models\tb_MOSSE_HDL_final\MOSSE%5FHDL%5Ffinal_DSP%5FBuilder%5FCompute%5FPSR_Psr1_Delay2.fixedpointlog  use_init=off  reset_value=1
  Divider : allblocks_alteradspbuilder2/Divider  BusType=Signed Integer  bwl=32  bwr=0  pipeline=0  pipeline_display=0  use_ena=off  use_aclr=off
  Multiplexer3 : allblocks_alteradspbuilder2/Multiplexer  numInputs=2  pipeline=0  oneHot=off  pipeline_display=0  use_ena=off  use_aclr=off  allowFloatingPointOverride=on  logOutputs=off  logFile=d:\Project\AutoTracking\model\MOSSE_work\MOSSE_model\MOSSE_Final_models\tb_MOSSE_HDL_final\MOSSE%5FHDL%5Ffinal_DSP%5FBuilder%5FCompute%5FPSR_Psr1_Multiplexer3.fixedpointlog
  Pipelined Adder : allblocks_alteradspbuilder2/Pipelined Adder  BusType=Signed Integer  bwl=32  bwr=0  pipeline=0  pipeline_display=0  AddSubDirection=SUB  use_cin=off  use_ovl=off  use_addsub=off  use_ena=off  use_aclr=off  or_aclr_inputs=on
  Psr_finish : Outport
  psr : Outport  Port=2
  wires:
  Pipelined Adder/1 -> Divider/1
  Divider/1 -> Multiplexer3/3
  max/1 -> Pipelined Adder/1
  mean/1 -> Pipelined Adder/2
  std/1 -> Divider/2
  psr_count_ena/1 -> Multiplexer3/1
  Multiplexer3/1 -> Delay2/1
  Delay2/1 -> psr/1, Multiplexer3/2
  std_finish/1 -> Delay1/1
  Delay1/1 -> Psr_finish/1

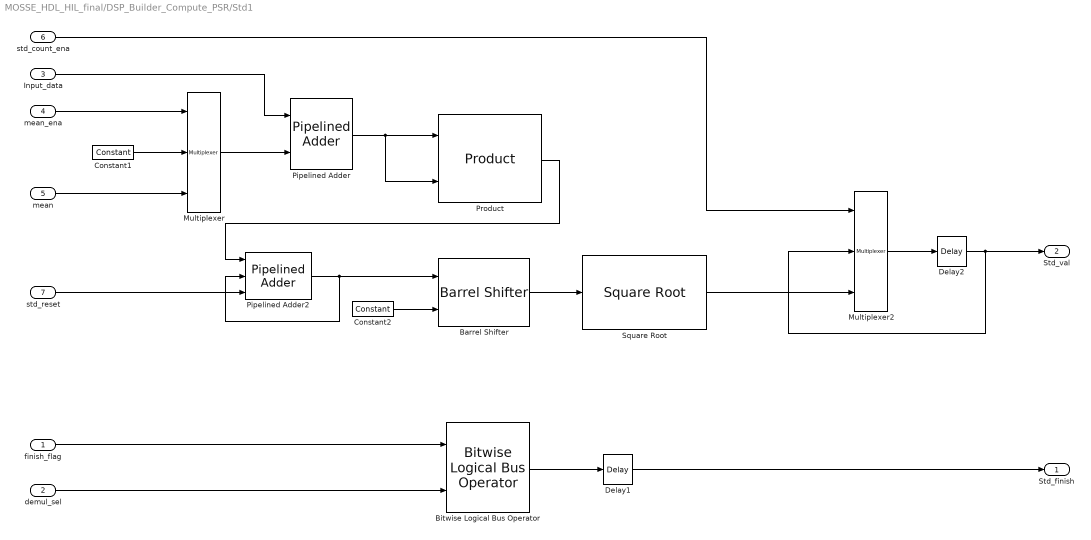
== system MOSSE_HDL_HIL_final/DSP_Builder_Compute_PSR/Std1 ==
  finish_flag : Inport
  demul_sel : Inport  Port=2
  Input_data : Inport  Port=3
  mean_ena : Inport  Port=4
  mean : Inport  Port=5
  std_count_ena : Inport  Port=6
  std_reset : Inport  Port=7
  Barrel Shifter : allblocks_alteradspbuilder2/Barrel Shifter  BusType=Signed Integer  bwl=44  bwr=8  pipeline=off  infer_distance=off  distance_length=4  ShiftDirection=Shift right  use_ena=off  use_aclr=off  UseDedicatedCircuitry=off  pipeline_display=0  allowFloatingPointOverride=on  logOutputs=off  logFile=d:\Project\AutoTracking\model\MOSSE_work\MOSSE_model\MOSSE_Final_models\tb_MOSSE_HDL_final\MOSSE%5FHDL%5Ffinal_DSP%5FBuilder%5FCompute%5FPSR_Std1_Barrel+Shifter.fixedpointlog
  Bitwise Logical Bus Operator : allblocks_alteradspbuilder2/Bitwise Logical Bus Operator  BusType=Unsigned Integer  bwl=1  bwr=0  LogicalOperator=AND  pipeline_display=0
  Constant1 : allblocks_alteradspbuilder2/Constant  mask_cst=0  BusType=Signed Integer  bwl=32  bwr=0  roundMode=Truncate  satMode=Wrap  SpecifyClock=off  allowFloatingPointOverride=on  logOutputs=off  logFile=d:\Project\AutoTracking\model\MOSSE_work\MOSSE_model\MOSSE_Final_models\tb_MOSSE_HDL_final\MOSSE%5FHDL%5Ffinal_DSP%5FBuilder%5FCompute%5FPSR_Std1_Constant1.fixedpointlog
  Constant2 : allblocks_alteradspbuilder2/Constant  mask_cst=12  BusType=Unsigned Integer  bwl=4  bwr=0  roundMode=Truncate  satMode=Wrap  SpecifyClock=off  allowFloatingPointOverride=on  logOutputs=off  logFile=d:\Project\AutoTracking\model\MOSSE_work\MOSSE_model\MOSSE_Final_models\tb_MOSSE_HDL_final\MOSSE%5FHDL%5Ffinal_DSP%5FBuilder%5FCompute%5FPSR_Std1_Constant2.fixedpointlog
  Delay1 : allblocks_alteradspbuilder2/Delay  pipeline=1  pipeline_display=1  ClockPhase=1  use_ena=off  use_sclr=off  allowFloatingPointOverride=on  logOutputs=off  logFile=d:\Project\AutoTracking\model\MOSSE_work\MOSSE_model\MOSSE_Final_models\tb_MOSSE_HDL_final\MOSSE%5FHDL%5Ffinal_DSP%5FBuilder%5FCompute%5FPSR_Std1_Delay1.fixedpointlog  use_init=off  reset_value=1
  Delay2 : allblocks_alteradspbuilder2/Delay  pipeline=1  pipeline_display=1  ClockPhase=1  use_ena=off  use_sclr=off  allowFloatingPointOverride=on  logOutputs=off  logFile=d:\Project\AutoTracking\model\MOSSE_work\MOSSE_model\MOSSE_Final_models\tb_MOSSE_HDL_final\MOSSE%5FHDL%5Ffinal_DSP%5FBuilder%5FCompute%5FPSR_Std1_Delay2.fixedpointlog  use_init=off  reset_value=1
  Multiplexer : allblocks_alteradspbuilder2/Multiplexer  numInputs=2  pipeline=0  oneHot=off  pipeline_display=0  use_ena=off  use_aclr=off  allowFloatingPointOverride=on  logOutputs=off  logFile=d:\Project\AutoTracking\model\MOSSE_work\MOSSE_model\MOSSE_Final_models\tb_MOSSE_HDL_final\MOSSE%5FHDL%5Ffinal_DSP%5FBuilder%5FCompute%5FPSR_Std1_Multiplexer.fixedpointlog
  Multiplexer2 : allblocks_alteradspbuilder2/Multiplexer  numInputs=2  pipeline=0  oneHot=off  pipeline_display=0  use_ena=off  use_aclr=off  allowFloatingPointOverride=on  logOutputs=off  logFile=d:\Project\AutoTracking\model\MOSSE_work\MOSSE_model\MOSSE_Final_models\tb_MOSSE_HDL_final\MOSSE%5FHDL%5Ffinal_DSP%5FBuilder%5FCompute%5FPSR_Std1_Multiplexer2.fixedpointlog
  Pipelined Adder : allblocks_alteradspbuilder2/Pipelined Adder  BusType=Signed Integer  bwl=32  bwr=0  pipeline=0  pipeline_display=0  AddSubDirection=SUB  use_cin=off  use_ovl=off  use_addsub=off  use_ena=off  use_aclr=off  or_aclr_inputs=on
  Pipelined Adder2 : allblocks_alteradspbuilder2/Pipelined Adder  BusType=Signed Integer  bwl=44  bwr=0  pipeline=1  pipeline_display=1  AddSubDirection=ADD  use_cin=off  use_ovl=off  use_addsub=off  use_ena=off  use_aclr=on  or_aclr_inputs=off
  Product : allblocks_alteradspbuilder2/Product  BusType=Signed Integer  bwl=32  bwr=0  pipeline=0  pipeline_display=0  phase_selection=1  use_ena=off  use_aclr=off  UseLPM=off  UseDedicatedCircuitry=on  allowFloatingPointOverride=on  logOutputs=off  logFile=d:\Project\AutoTracking\model\MOSSE_work\MOSSE_model\MOSSE_Final_models\tb_MOSSE_HDL_final\MOSSE%5FHDL%5Ffinal_DSP%5FBuilder%5FCompute%5FPSR_Std1_Product.fixedpointlog
  Square Root : allblocks_alteradspbuilder2/Square Root  BusType=Unsigned Integer  bwl=44  bwr=0  pipeline=0  pipeline_display=0  use_remain=off  use_ena=off  use_aclr=off
  Std_finish : Outport
  Std_val : Outport  Port=2
  wires:
  Pipelined Adder/1 -> Product/2, Product/1
  Product/1 -> Pipelined Adder2/1
  Constant2/1 -> Barrel Shifter/2
  Pipelined Adder2/1 -> Pipelined Adder2/2, Barrel Shifter/1
  Barrel Shifter/1 -> Square Root/1
  Square Root/1 -> Multiplexer2/3
  Input_data/1 -> Pipelined Adder/1
  demul_sel/1 -> Bitwise Logical Bus Operator/2
  finish_flag/1 -> Bitwise Logical Bus Operator/1
  Delay1/1 -> Std_finish/1
  Constant1/1 -> Multiplexer/2
  mean_ena/1 -> Multiplexer/1
  mean/1 -> Multiplexer/3
  Multiplexer/1 -> Pipelined Adder/2
  std_count_ena/1 -> Multiplexer2/1
  Multiplexer2/1 -> Delay2/1
  Delay2/1 -> Std_val/1, Multiplexer2/2
  Bitwise Logical Bus Operator/1 -> Delay1/1
  std_reset/1 -> Pipelined Adder2/3

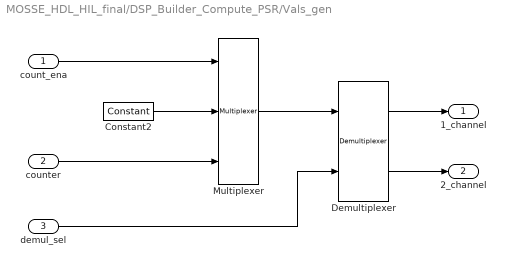
== system MOSSE_HDL_HIL_final/DSP_Builder_Compute_PSR/Vals_gen ==
  count_ena : Inport
  counter : Inport  Port=2
  demul_sel : Inport  Port=3
  Constant2 : allblocks_alteradspbuilder2/Constant  mask_cst=0  BusType=Single Bit  bwl=16  bwr=0  roundMode=Truncate  satMode=Wrap  SpecifyClock=off  allowFloatingPointOverride=on  logOutputs=off  logFile=d:\Project\AutoTracking\model\MOSSE_work\MOSSE_model\MOSSE_Final_models\tb_MOSSE_HDL_final\MOSSE%5FHDL%5Ffinal_DSP%5FBuilder%5FCompute%5FPSR_Vals%5Fgen_Constant2.fixedpointlog
  Demultiplexer : allblocks_alteradspbuilder2/Demultiplexer  numOutputs=2  pipeline_display=1  use_ena=off  use_sclr=off  allowFloatingPointOverride=on  logOutputs=off  logFile=d:\Project\AutoTracking\model\MOSSE_work\MOSSE_model\MOSSE_Final_models\tb_MOSSE_HDL_final\MOSSE%5FHDL%5Ffinal_DSP%5FBuilder%5FCompute%5FPSR_Vals%5Fgen_Demultiplexer%3A%3Aq.fixedpointlog,d:\Project\AutoTracking\model\MOSSE_work\MOSSE_model\MOSSE_Final_models\tb_MOSSE_HDL_final\MOSSE%5FHDL%5Ffinal_DSP%5FBuilder%5FCompute%5FPSR_Vals%5Fgen_Demultiplexer%3A%3Aq.fixedpointlog,
  Multiplexer : allblocks_alteradspbuilder2/Multiplexer  numInputs=2  pipeline=0  oneHot=off  pipeline_display=0  use_ena=off  use_aclr=off  allowFloatingPointOverride=on  logOutputs=off  logFile=d:\Project\AutoTracking\model\MOSSE_work\MOSSE_model\MOSSE_Final_models\tb_MOSSE_HDL_final\MOSSE%5FHDL%5Ffinal_DSP%5FBuilder%5FCompute%5FPSR_Vals%5Fgen_Multiplexer.fixedpointlog
  1_channel : Outport
  2_channel : Outport  Port=2
  wires:
  Multiplexer/1 -> Demultiplexer/1
  Demultiplexer/1 -> 1_channel/1
  Demultiplexer/2 -> 2_channel/1
  demul_sel/1 -> Demultiplexer/2
  Constant2/1 -> Multiplexer/2
  counter/1 -> Multiplexer/3
  count_ena/1 -> Multiplexer/1

== system MOSSE_HDL_HIL_final/Source/source_1 ==
  In1 : Inport
  Enable : EnablePort
  source_1 : LookupNDDirect  NumberOfTableDimensions=1  Table=source_1  TableDataTypeStr=int16
  Out1 : Outport
  wires:
  source_1/1 -> Out1/1
  In1/1 -> source_1/1

== system MOSSE_HDL_HIL_final/Source/source_2 ==
  In1 : Inport
  Enable : EnablePort
  source_2 : LookupNDDirect  NumberOfTableDimensions=1  Table=source_2  TableDataTypeStr=int16
  Out1 : Outport
  wires:
  source_2/1 -> Out1/1
  In1/1 -> source_2/1

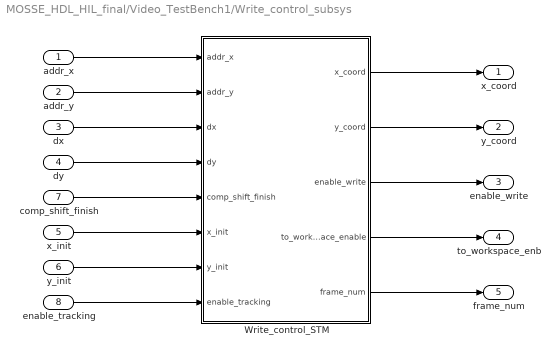
== system MOSSE_HDL_HIL_final/Video_TestBench1/Write_control_subsys ==
  addr_x : Inport
  addr_y : Inport  Port=2
  dx : Inport  Port=3
  dy : Inport  Port=4
  x_init : Inport  Port=5
  y_init : Inport  Port=6
  comp_shift_finish : Inport  Port=7
  enable_tracking : Inport  Port=8
  Write_control_STM : State Transition Table  TreatAsAtomicUnit=on
  x_coord : Outport
  y_coord : Outport  Port=2
  enable_write : Outport  Port=3
  to_workspace_enb : Outport  Port=4
  frame_num : Outport  Port=5
  wires:
  x_init/1 -> Write_control_STM/6(x_init)
  y_init/1 -> Write_control_STM/7(y_init)
  dx/1 -> Write_control_STM/3(dx)
  dy/1 -> Write_control_STM/4(dy)
  Write_control_STM/1(x_coord) -> x_coord/1
  Write_control_STM/3(enable_write) -> enable_write/1
  Write_control_STM/2(y_coord) -> y_coord/1
  comp_shift_finish/1 -> Write_control_STM/5(comp_shift_finish)
  Write_control_STM/4(to_workspace_enable) -> to_workspace_enb/1
  addr_x/1 -> Write_control_STM/1(addr_x)
  addr_y/1 -> Write_control_STM/2(addr_y)
  Write_control_STM/5(frame_num) -> frame_num/1
  enable_tracking/1 -> Write_control_STM/8(enable_tracking)

== system MOSSE_HDL_HIL_final/Video_TestBench1/deserialize1 ==
  serialin : Inport
  Buffer : Buffer  N=640*360  TreatMby1Signals=One channel
  Convert 1-D to 2-D : dspsigattribs/Convert 1-D to 2-D  M=640  N=360  frameBasedOut=off
  Frame Conversion : FrameConversion  OutFrame=Sample-based
  Transpose : dspmtrx3/Transpose  Hermitian=off  overflowFlag=on
  imgout : Outport
  wires:
  Buffer/1 -> Frame Conversion/1
  serialin/1 -> Buffer/1
  Convert 1-D to 2-D/1 -> Transpose/1
  Frame Conversion/1 -> Convert 1-D to 2-D/1
  Transpose/1 -> imgout/1

== system MOSSE_HDL_HIL_final/Video_TestBench1/serialize ==
  img : Inport
  Convert 2-D to 1-D : dspsigattribs/Convert 2-D to 1-D
  Frame Conversion : FrameConversion
  Transpose : dspmtrx3/Transpose  Hermitian=off  overflowFlag=on
  Unbuffer : Unbuffer  SampleBasedProcessing=Same as frame based
  serial : Outport  SampleTime=1
  wires:
  Convert 2-D to 1-D/1 -> Frame Conversion/1
  img/1 -> Transpose/1
  Transpose/1 -> Convert 2-D to 1-D/1
  Frame Conversion/1 -> Unbuffer/1
  Unbuffer/1 -> serial/1

== stateflow chart Source/State Transition Table ==
  state state2
    entry:
    enable_write = false;
  state state1
    entry:
    enable_write = false;
  state state3
    entry:
    enable_write = true;
  state state4
    entry:
    enable_write = false;
  state1 -> (junction 27) [order 2]
  (default) -> state1
  (junction 27) -> state1
  state1 -> state2 [order 1] : {temp = 0;
      | count = 0;}
  state2 -> (junction 28) [order 2]
  (junction 28) -> state2
  (junction 29) -> state2
  (junction 32) -> (junction 29)
  state2 -> state3 [order 1] : [address == 99541 + temp*640]
  state3 -> (junction 30) [order 1] : [count ~= 127]
      | {count = count + 1;}
  (junction 30) -> state3
  state3 -> state4 [order 2] : {temp = temp + 1;
      |  count = 0;}
  state4 -> (junction 31) [order 2] : {temp = 0;}
  (junction 31) -> state4
  state4 -> (junction 32) [order 1] : [temp ~= 128]
  data: enable_write output boolean; address input uint32; temp local double; count local double
